simulink model "turbine_Drivetrain_modelling"  (R2024a)
settings: Solver=VariableStepAuto  StartTime=0.0  StopTime=200  MaxStep=0.4  RelTol=1e-3
model workspace (MAT data in the model file):
  para_mdl = Simulink.Parameter
  para_mdl.Value.N = 3
  para_mdl.Value.R = 63
  para_mdl.Value.rho = 1.225
  para_mdl.Value.mT = 436865
  para_mdl.Value.kT = 1981900
  para_mdl.Value.dT = 70000
  para_mdl.Value.rB = 21.975
  para_mdl.Value.mB = 4435
  para_mdl.Value.kB = 40000
  para_mdl.Value.kB_zentr = 0.02
  para_mdl.Value.dB = 20000
  para_mdl.Value.ngear = 97
  para_mdl.Value.Jr = 38759227
  para_mdl.Value.Jg = 534.1
  para_mdl.Value.kS = 92213.5189712
  para_mdl.Value.dS = 660.537782974
  para_mdl.Value.tau_beta = 0.1
  para_mdl.Value.betaP_max = 0.174532925199
  para_mdl.Value.tau_PT2 = 0.09
  para_mdl.Value.zeta_PT2 = 0.6
  para_mdl.Value.tau_g = 0.02
  para_mdl.Value.Tv = 4
  para_mdl.Value.Notch.om1 = 10.364
  para_mdl.Value.Notch.om2 = 8
  para_mdl.Value.Notch.zeta1 = 0.6
  para_mdl.Value.Notch.zeta2 = 1.2
  para_mdl.Value.Pr_R = 5296610
  para_mdl.Value.omega_r_R = 1.2671
  para_mdl.Value.omega_g_R = 122.9087
  para_mdl.Value.Tr_R = 4180104.17489
  para_mdl.Value.Tg_R = 43093.8574731
  para_mdl.Value.v_R = 11.26
  para_mdl.Value.J_1DOF = 43784573.9
  para_mdl.Value.CT_betas = [0 0.0872664625997 0.174532925199 0.261799387799 0.349065850399 0.436332312999 0.523598775598 0.698131700798 0.872664625997 1.0471975512 1.2217304764 1.3962634016 1.57079632679]
  para_mdl.Value.CT_lambdas = [0; 0.25; 0.5; 0.75; 1; 1.25; 1.5; 2; 2.5; 3; 3.5; 4; 4.5; 5; 5.5; 6; 6.5; 7; 7.5; 8; 8.5; 9; 9.5; 10; 10.5; 11; 11.5; 12; 12.5; 13; 13.5; 14; 14.5; 15; 15.5; 16; 16.5; 17; 17.5]
  para_mdl.Value.CQ_betas = [0 0.0872664625997 0.174532925199 0.261799387799 0.349065850399 0.436332312999 0.523598775598 0.698131700798 0.872664625997 1.0471975512 1.2217304764 1.3962634016 1.57079632679]
  para_mdl.Value.CQ_lambdas = [0; 0.25; 0.5; 0.75; 1; 1.25; 1.5; 2; 2.5; 3; 3.5; 4; 4.5; 5; 5.5; 6; 6.5; 7; 7.5; 8; 8.5; 9; 9.5; 10; 10.5; 11; 11.5; 12; 12.5; 13; 13.5; 14; 14.5; 15; 15.5; 16; 16.5; 17; 17.5]
  para_mdl.Value.CQ_entries = [0.00463492513935 0.0049015417371 0.00516815833485 0.00555696036228 0.0059457623897 0.00611397686765 0.00628219134561 0.012914252991 0.0255245334589 0.0349006692545 0.0430149587943 0.0524658396931 ... (507 elements, 39x13)]
  para_mdl.Value.CT_entries = [0.0686211548678 0.0728422059393 0.0770632570108 0.0836290674204 0.09019487783 0.0932108047116 0.0962267315932 0.135717354129 0.192838891055 0.239446349533 0.288110808378 0.351656989082 ... (507 elements, 39x13)]
  para_mdl.Value.Cp_max = 0.487647762952
  para_mdl.Value.lambda_opt = 7.5
  para_mdl.Complexity = 'real'
  para_mdl.Dimensions = [1 1]
  para_mdl.DataType = 'struct'
values from neighbouring files (symbols this model uses):
  beta = [0.0000, 0.0306, 0.0560, 0.0772, 0.0953, 0.1113, 0.1254, 0.1382,          0.1499, 0.1607, 0.1783, 0.2134, 0.2421, 0.2669, 0.2890, 0.3091,          0.3279, 0.3456, 0.3625, 0.3789]'    [Sensitivities.m]
  k_I = a./(b.*tau_ref)    [Sensitivities.m]
  k_P = 5./(b.*tau_ref)    [Sensitivities.m]
  para_mdl =     [para_mdl_WT_with_aero.mat]
  v = [11.2600, 11.5378, 11.8156, 12.0933, 12.3711, 12.6489, 12.9267,       13.2044, 13.4822, 13.7600, 14.2600, 15.4533, 16.6467, 17.8400,       19.0333, 20.2267, 21.4200, 22.6133, 23.8067, 25.0000]'    [Sensitivities.m]
settings Model: Creator=hasansinat  LastModifiedBy=Dell
settings SolverCC: AlgebraicLoopSolver=TrustRegion
settings RTWCC: GPUComputeCapability=3.5

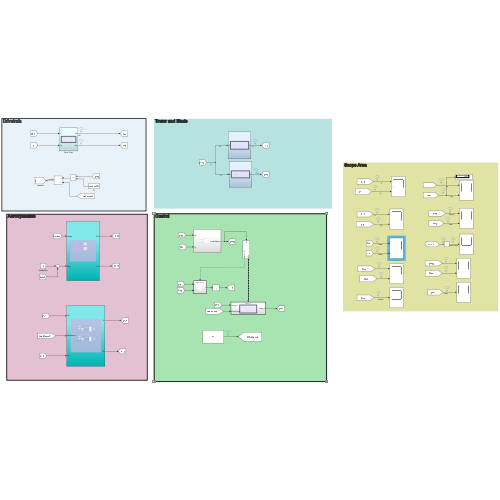
[thumbnail: Simulink's stored preview of the top-level diagram]
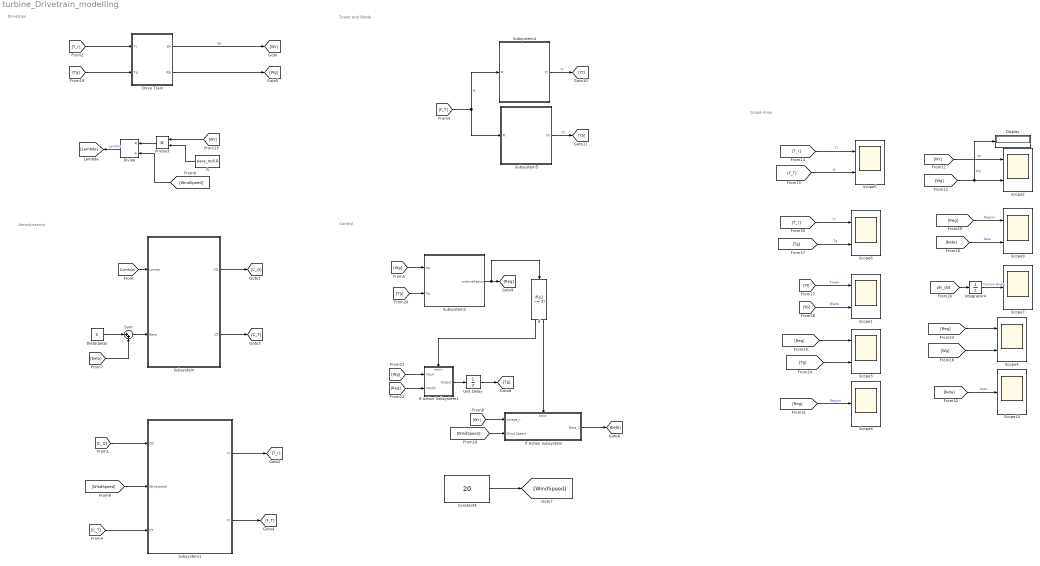
== system turbine_Drivetrain_modelling ==
  note: Aerodynamics
  note: Drivetrain
  note: Tower and Blade
  note: Control
  note: Scope Area
  Constant4 : Constant  Value=20
  Display : Display
  Divide : Product  Inputs=*/
  Drive Train : Subsystem
  If : If  IfExpression=u1 ~= 3
  If Action Subsystem : Subsystem  TreatAsAtomicUnit=on
  If Action Subsystem1 : Subsystem  TreatAsAtomicUnit=on
  Integrator4 : Integrator
  Product : Product
  R : Constant  Value=para_mdl.R
  Scope{1..6,9} (7 alike) : Scope  NumInputPorts=2
  Scope10 : Scope
  Scope7 : Scope
  Scope8 : Scope
  Subsystem : Subsystem
  Subsystem1 : Subsystem
  Subsystem2 : Subsystem
  Subsystem4 : Subsystem
  Subsystem5 : Subsystem
  Sum : Sum  Inputs=|++
  Unit Delay : UnitDelay  SampleTime=-1  HasFrameUpgradeWarning=on
  theta(beta) : Constant  Value=0
  wires:
  [T_r] -> Drive Train/1(Tr)
  Drive Train/1(Wr) -> [Wr]  "Wr"
  Product/1 -> Divide/1
  R/1 -> Product/2
  Divide/1 -> [Lambda]  "Lambda"
  Drive Train/2(Wg) -> [Wg]
  Unit Delay/1 -> [Tg]
  If/2 -> If Action Subsystem/Action
  If/1 -> If Action Subsystem1/Action
  If Action Subsystem/1(Beta_1) -> [beta]
  theta(beta)/1 -> Sum/1
  [Wr] -> If Action Subsystem/1(omega_r)
  [WindSpeed] -> If Action Subsystem/2(Wind Speed)
  [Wr] -> Scope2/1  "Wr"
  [Wg] -> Display/1, Scope2/2  "Wg"
  [Wr] -> Product/1
  [T_r] -> Scope5/1  "Tr"
  [F_T] -> Scope5/2  "Ft"
  [beta] -> Scope9/2  "beta"
  [Tg] -> Scope6/2  "Tg"
  [beta] -> Sum/2
  If Action Subsystem1/1(Output) -> Unit Delay/1
  [Wg] -> Scope4/2
  [Tg] -> Drive Train/2(Tg)
  [Wg] -> If Action Subsystem1/1(Input)
  [Reg] -> If Action Subsystem1/2(Input1)
  [Reg] -> Scope4/1
  [Tg] -> Scope3/2
  [Reg] -> Scope3/1
  [Lambda] -> Subsystem/1(Lamda)
  Sum/1 -> Subsystem/2(Beta)
  Subsystem/1(CQ) -> [C_Q]
  Subsystem/2(CT) -> [C_T]
  [C_Q] -> Subsystem1/1(CQ)
  [WindSpeed] -> Subsystem1/2(Windspeed)
  [C_T] -> Subsystem1/3(CT)
  Subsystem1/1(Tr) -> [T_r]
  Subsystem1/2(Ft) -> [F_T]
  Subsystem5/1(Yb) -> [Yb]  "Yb"
  [F_T] -> Subsystem5/1(Ft), Subsystem4/1(Ft)  "Ft"
  Subsystem4/1(Yt) -> [Yt]  "Yt"
  Subsystem2/1(turbineRegion) -> If/1, [Reg]
  [Wg] -> Subsystem2/1(wg)
  [Tg] -> Subsystem2/2(Tg)
  [phi_dot] -> Integrator4/1
  Integrator4/1 -> Scope7/1  "Torsion Angle"
  [Yb] -> Scope1/2  "Blade"
  [Yt] -> Scope1/1  "Tower"
  Constant4/1 -> [WindSpeed]
  [WindSpeed] -> Divide/2
  [Reg] -> Scope9/1  "Region"
  [T_r] -> Scope6/1  "Tr"
  [Reg] -> Scope8/1  "Region"
  [beta] -> Scope10/1  "beta"

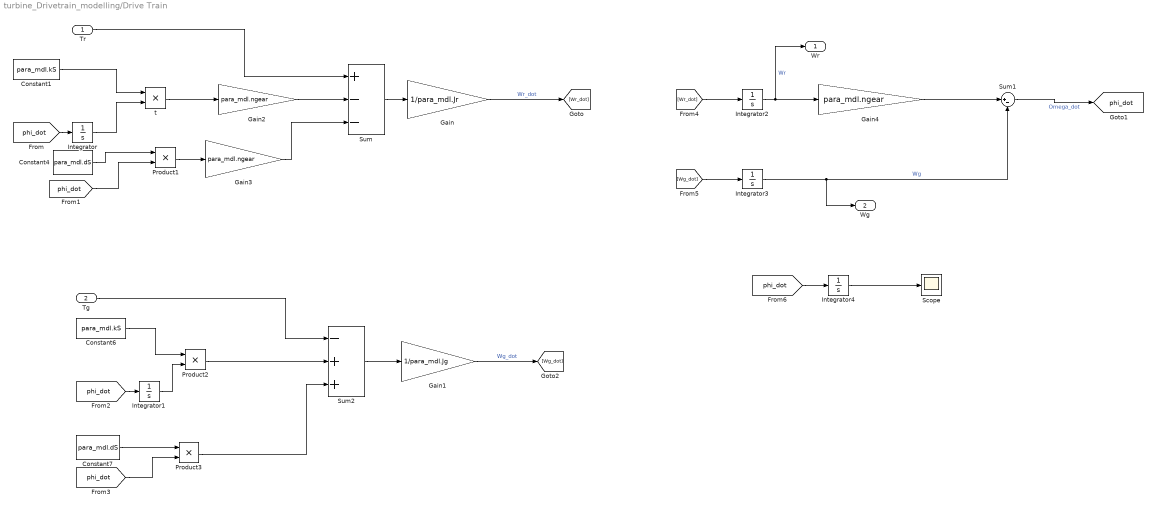
== system turbine_Drivetrain_modelling/Drive Train ==
  Tr : Inport
  Tg : Inport  Port=2
  Constant1 : Constant  Value=para_mdl.kS
  Constant4 : Constant  Value=para_mdl.dS
  Constant6 : Constant  Value=para_mdl.kS
  Constant7 : Constant  Value=para_mdl.dS
  Gain : Gain  Gain=1/para_mdl.Jr
  Gain1 : Gain  Gain=1/para_mdl.Jg
  Gain2 : Gain  Gain=para_mdl.ngear
  Gain3 : Gain  Gain=para_mdl.ngear
  Gain4 : Gain  Gain=para_mdl.ngear
  Integrator{,1..4} (5 alike) : Integrator
  Product1 : Product
  Product2 : Product
  Product3 : Product
  Scope : Scope
  Sum : Sum  Inputs=+--
  Sum1 : Sum  Inputs=|+-
  Sum2 : Sum  Inputs=-++
  t : Product
  Wr : Outport
  Wg : Outport  Port=2
  tag scope: phi_dot=global
  wires:
  [Wr_dot] -> Integrator2/1
  Gain4/1 -> Sum1/1
  [phi_dot] -> Integrator1/1
  Constant4/1 -> Product1/1
  Integrator2/1 -> Wr/1, Gain4/1  "Wr"
  Constant6/1 -> Product2/1
  Tg/1 -> Sum2/1
  Sum1/1 -> [phi_dot]  "Omega_dot"
  Constant7/1 -> Product3/1
  Integrator3/1 -> Wg/1, Sum1/2  "Wg"
  Sum/1 -> Gain/1
  Sum2/1 -> Gain1/1
  [phi_dot] -> Product3/2
  Gain1/1 -> [Wg_dot]  "Wg_dot"
  Constant1/1 -> t/1
  [phi_dot] -> Product1/2
  [phi_dot] -> Integrator/1
  Integrator1/1 -> Product2/2
  Integrator/1 -> t/2
  [Wg_dot] -> Integrator3/1
  Gain/1 -> [Wr_dot]  "Wr_dot"
  Tr/1 -> Sum/1
  t/1 -> Gain2/1
  Product2/1 -> Sum2/2
  Product3/1 -> Sum2/3
  Gain2/1 -> Sum/2
  Gain3/1 -> Sum/3
  [phi_dot] -> Integrator4/1
  Integrator4/1 -> Scope/1
  Product1/1 -> Gain3/1

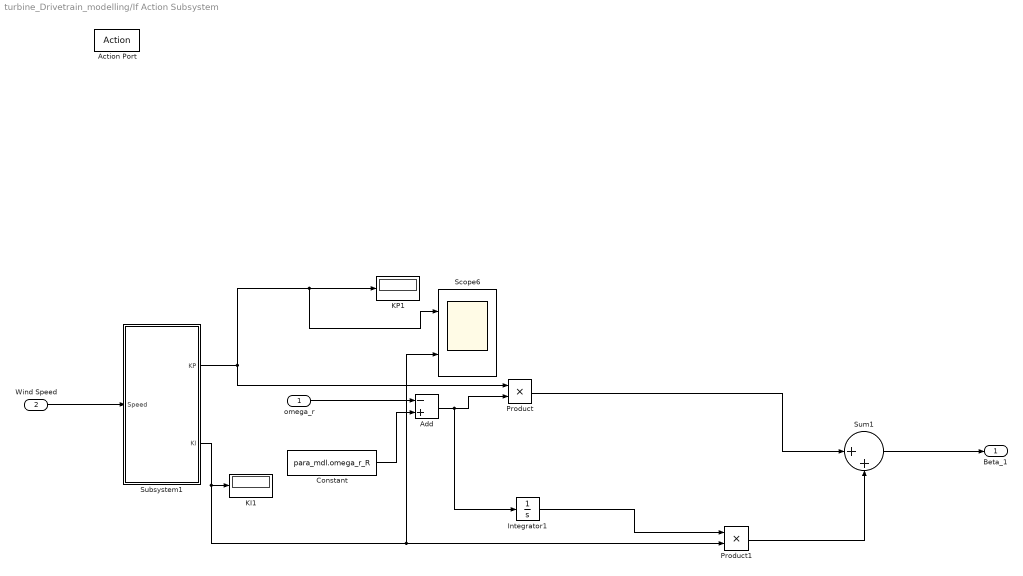
== system turbine_Drivetrain_modelling/If Action Subsystem ==
  omega_r : Inport
  Wind Speed : Inport  Port=2
  Action Port : ActionPort  ActionPortLabel=else
  Add : Sum  Inputs=-+
  Constant : Constant  Value=para_mdl.omega_r_R
  Integrator1 : Integrator
  KI1 : Display
  KP1 : Display
  Product : Product
  Product1 : Product
  Scope6 : Scope  NumInputPorts=2
  Subsystem1 : Subsystem  Priority=1
  Sum1 : Sum  Inputs=|++
  Beta_1 : Outport
  wires:
  Constant/1 -> Add/2
  Integrator1/1 -> Product1/1
  Add/1 -> Integrator1/1, Product/2
  Product/1 -> Sum1/1
  Wind Speed/1 -> Subsystem1/1(Speed)
  Sum1/1 -> Beta_1/1
  Subsystem1/2(" KI") -> Scope6/2, Product1/2, KI1/1
  Subsystem1/1(" KP") -> Scope6/1, KP1/1, Product/1
  omega_r/1 -> Add/1
  Product1/1 -> Sum1/2

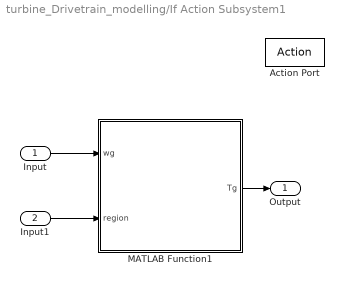
== system turbine_Drivetrain_modelling/If Action Subsystem1 ==
  Input : Inport
  Input1 : Inport  Port=2
  Action Port : ActionPort  ActionPortLabel=if(u1 ~= 3)
  MATLAB Function1 : MATLAB Function  TreatAsAtomicUnit=on
  Output : Outport
  wires:
  Input1/1 -> MATLAB Function1/2(region)
  Input/1 -> MATLAB Function1/1(wg)
  MATLAB Function1/1(Tg) -> Output/1

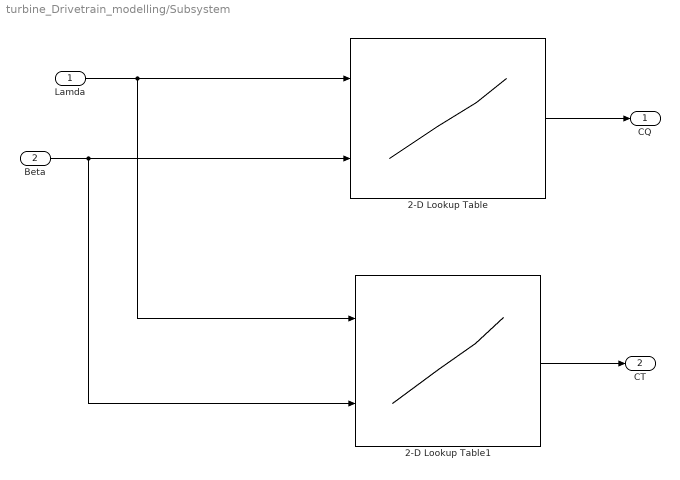
== system turbine_Drivetrain_modelling/Subsystem ==
  Lamda : Inport
  Beta : Inport  Port=2
  2-D Lookup Table : Lookup_n-D  BreakpointsForDimension1=para_mdl.CQ_lambdas  BreakpointsForDimension2=para_mdl.CQ_betas  Table=para_mdl.CQ_entries  InternalRulePriority=Speed  RndMeth=Simplest
      settings: InputPortMap=u0,u1
  2-D Lookup Table1 : Lookup_n-D  BreakpointsForDimension1=para_mdl.CT_lambdas  BreakpointsForDimension2=para_mdl.CT_betas  Table=para_mdl.CT_entries  InternalRulePriority=Speed  RndMeth=Simplest
      settings: InputPortMap=u0,u1
  CQ : Outport
  CT : Outport  Port=2
  wires:
  Beta/1 -> 2-D Lookup Table/2, 2-D Lookup Table1/2
  2-D Lookup Table1/1 -> CT/1
  Lamda/1 -> 2-D Lookup Table1/1, 2-D Lookup Table/1
  2-D Lookup Table/1 -> CQ/1

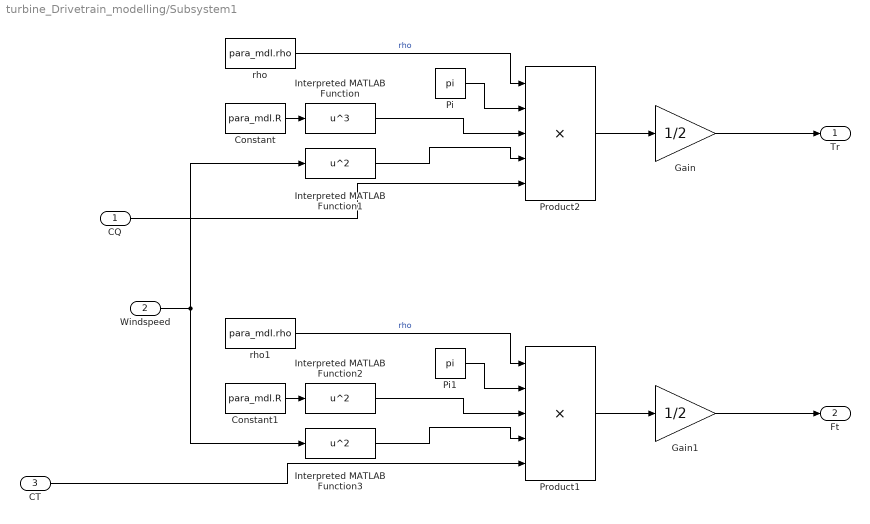
== system turbine_Drivetrain_modelling/Subsystem1 ==
  CQ : Inport
  Windspeed : Inport  Port=2
  CT : Inport  Port=3
  Constant : Constant  Value=para_mdl.R
  Constant1 : Constant  Value=para_mdl.R
  Gain : Gain  Gain=1/2
  Gain1 : Gain  Gain=1/2
  Interpreted MATLAB Function : MATLABFcn  MATLABFcn=u^3
  Interpreted MATLAB Function1 : MATLABFcn  MATLABFcn=u^2
  Interpreted MATLAB Function2 : MATLABFcn  MATLABFcn=u^2
  Interpreted MATLAB Function3 : MATLABFcn  MATLABFcn=u^2
  Pi : Constant  Value=pi  OutDataTypeStr=Inherit: Inherit via back propagation
  Pi1 : Constant  Value=pi  OutDataTypeStr=Inherit: Inherit via back propagation
  Product1 : Product  Inputs=5
  Product2 : Product  Inputs=5
  rho : Constant  Value=para_mdl.rho
  rho1 : Constant  Value=para_mdl.rho
  Tr : Outport
  Ft : Outport  Port=2
  wires:
  Product2/1 -> Gain/1
  Windspeed/1 -> Interpreted MATLAB Function1/1, Interpreted MATLAB Function3/1
  Product1/1 -> Gain1/1
  Pi/1 -> Product2/2
  Interpreted MATLAB Function1/1 -> Product2/4
  Pi1/1 -> Product1/2
  Interpreted MATLAB Function3/1 -> Product1/4
  Gain/1 -> Tr/1
  Constant/1 -> Interpreted MATLAB Function/1
  Gain1/1 -> Ft/1
  Constant1/1 -> Interpreted MATLAB Function2/1
  Interpreted MATLAB Function2/1 -> Product1/3
  rho/1 -> Product2/1  "rho"
  Interpreted MATLAB Function/1 -> Product2/3
  rho1/1 -> Product1/1  "rho"
  CQ/1 -> Product2/5
  CT/1 -> Product1/5

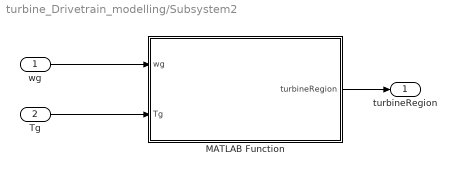
== system turbine_Drivetrain_modelling/Subsystem2 ==
  wg : Inport
  Tg : Inport  Port=2
  MATLAB Function : MATLAB Function  TreatAsAtomicUnit=on
  turbineRegion : Outport
  wires:
  wg/1 -> MATLAB Function/1(wg)
  Tg/1 -> MATLAB Function/2(Tg)
  MATLAB Function/1(turbineRegion) -> turbineRegion/1

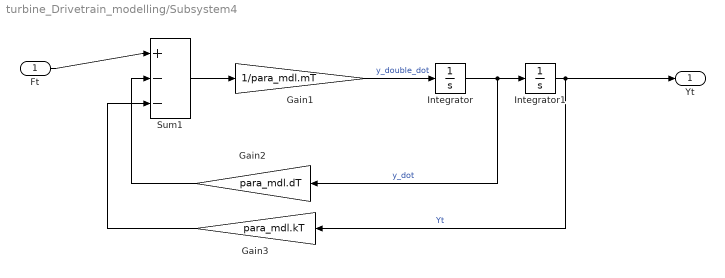
== system turbine_Drivetrain_modelling/Subsystem4 ==
  Ft : Inport
  Gain1 : Gain  Gain=1/para_mdl.mT
  Gain2 : Gain  Gain=para_mdl.dT
  Gain3 : Gain  Gain=para_mdl.kT
  Integrator : Integrator
  Integrator1 : Integrator
  Sum1 : Sum  Inputs=|+--
  Yt : Outport
  wires:
  Sum1/1 -> Gain1/1
  Ft/1 -> Sum1/1
  Integrator1/1 -> Yt/1, Gain3/1  "Yt"
  Gain2/1 -> Sum1/2
  Gain1/1 -> Integrator/1  "y_double_dot"
  Gain3/1 -> Sum1/3
  Integrator/1 -> Integrator1/1, Gain2/1  "y_dot"

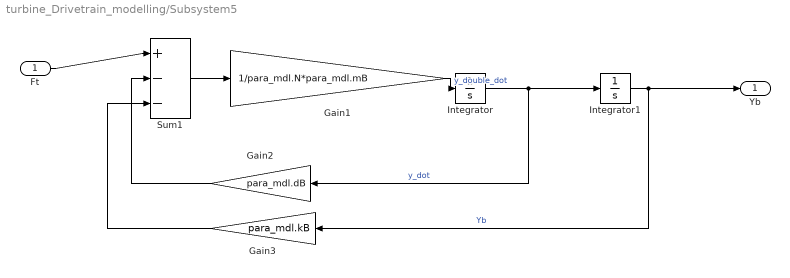
== system turbine_Drivetrain_modelling/Subsystem5 ==
  Ft : Inport
  Gain1 : Gain  Gain=1/para_mdl.N*para_mdl.mB
  Gain2 : Gain  Gain=para_mdl.dB
  Gain3 : Gain  Gain=para_mdl.kB
  Integrator : Integrator
  Integrator1 : Integrator
  Sum1 : Sum  Inputs=|+--
  Yb : Outport
  wires:
  Integrator/1 -> Integrator1/1, Gain2/1  "y_dot"
  Gain3/1 -> Sum1/3
  Gain1/1 -> Integrator/1  "y_double_dot"
  Gain2/1 -> Sum1/2
  Integrator1/1 -> Yb/1, Gain3/1  "Yb"
  Ft/1 -> Sum1/1
  Sum1/1 -> Gain1/1

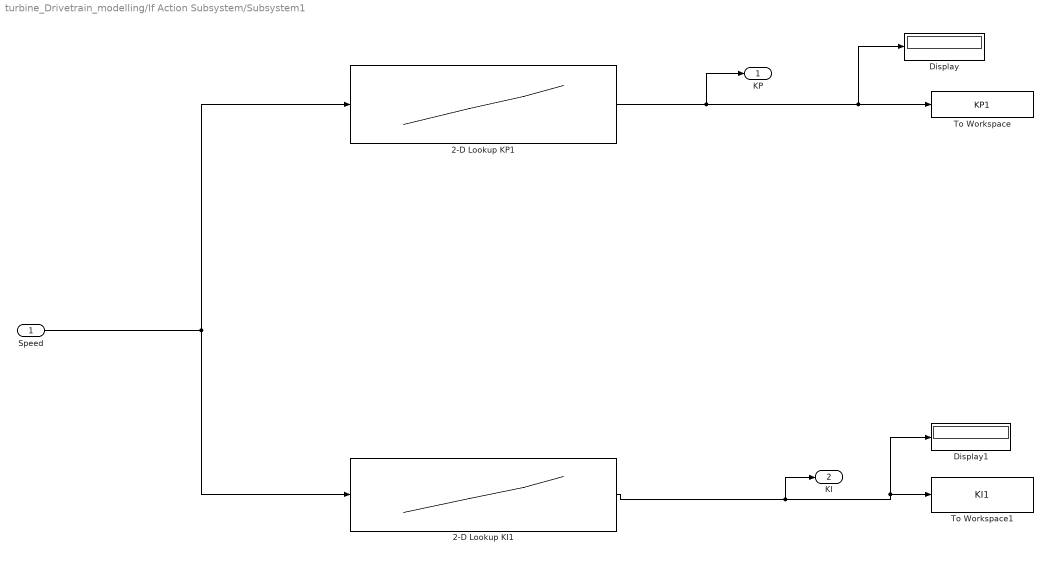
== system turbine_Drivetrain_modelling/If Action Subsystem/Subsystem1 ==
  Speed : Inport
  2-D Lookup KI1 : Lookup_n-D  NumberOfTableDimensions=1  BreakpointsForDimension1=v  BreakpointsForDimension2=beta  Table=k_I  InternalRulePriority=Speed  RndMeth=Simplest
  2-D Lookup KP1 : Lookup_n-D  NumberOfTableDimensions=1  BreakpointsForDimension1=v  BreakpointsForDimension2=[1:3]  Table=k_P  InternalRulePriority=Speed  RndMeth=Simplest
  Display : Display
  Display1 : Display
  To Workspace : ToWorkspace  VariableName=KP1  SaveFormat=Timeseries  SampleTime=-1
  To Workspace1 : ToWorkspace  VariableName=KI1  SaveFormat=Timeseries  SampleTime=-1
  " KP" : Outport
  " KI" : Outport  Port=2
  wires:
  2-D Lookup KI1/1 -> " KI"/1, Display1/1, To Workspace1/1
  Speed/1 -> 2-D Lookup KP1/1, 2-D Lookup KI1/1
  2-D Lookup KP1/1 -> " KP"/1, Display/1, To Workspace/1

== matlab function turbine_Drivetrain_modelling/Subsystem2/MATLAB Function ==
  settings: updateMethod=DISCRETE
  data: wg input; turbineRegion output; Tg input
function turbineRegion = fcn(wg, Tg)
    %#codegen

    % Define the thresholds for the conditions
    wg_rated = 1.229087000000000e+02;
    wg_R1_max = wg_rated * 0.5708; 
    wg_R1_5_max = wg_rated * 0.7421;
    wg_R2_max = wg_rated * 0.9782;
    wg_R2_5_max = wg_rated * 0.99;
     
    dwg = 2;
    Tg_max = 4.309385747306741e+04;

    % Define a persistent variable to store the previous region
    persistent prev_region
    if isempty(prev_region)
        prev_region = 1; % initialize with the starting region
    end
    % Declare that prev_region can have a variable size
    coder.varsize('prev_region', [1, 5], [0, 1]); % [1, 5] is the maximum size, [0, 1] indicates that the second dimension can vary

    % Initialize the region output
    turbineRegion = 0;
    % Check the conditions for each region
    switch prev_region
        case 1 % Region_1
            if wg > wg_R1_max
                turbineRegion = 1.5; % Region_1.5
            else
                turbineRegion = 1; % Region_1
            end
        case 2 % Region_1.5
            if wg > wg_R1_5_max
                turbineRegion = 2; % Region_2
            elseif wg <= wg_R1_max
                turbineRegion = 1; % Region_1
            else
                turbineRegion = 1.5; % Region_1.5
            end
        case 3 % Region_2
            if wg > wg_R2_max && Tg > Tg_max
                turbineRegion = 2.5; % Region_2.5
            elseif wg <= wg_R1_5_max
                turbineRegion = 1.5; % Region_1.5
            else
                turbineRegion = 2; % Region_2
            end
        case 4 % Region_2.5
            if wg > wg_R2_5_max && Tg > Tg_max
                turbineRegion = 3; % Region_3
            elseif wg <= (wg_R2_max - dwg)
                turbineRegion = 2; % Region_2
            else
                turbineRegion = 2.5; % Region_2.5
            end
        case 5 % Region_3
            if wg <= wg_R2_5_max || Tg <= Tg_max
                turbineRegion = 2.5; % Region_2.5
            else
                turbineRegion = 3; % Region_3
            end
    end

    % Update the previous region
    prev_region = find([1, 1.5, 2, 2.5, 3] == turbineRegion);
end

== matlab function turbine_Drivetrain_modelling/If Action Subsystem1/MATLAB Function1 ==
  data: wg input; Tg output; region input
function Tg = calculateTg(wg, region)
    % Calculation for Tg based on operating region

    wg_rated = 1.229087000000000e+02;
    Tg_max = 4.309385747306741e+04;
    k_Opt = 2.418610624349642;
    %k_Opt = 0.5 * 1.2250 * pi * 63^5 * (0.4876/(97^3*7.5^3)) * wg^2;
    
    switch region
        case 1
            Tg = 0; % Region 1
        case 1.5
            Tg = (3*(wg/wg_rated) - 1.8)*Tg_max; % Region 1.5
        case 2
            Tg = k_Opt * wg^2; % Region 2
        case 2.5
            Tg = (5.5*(wg/wg_rated) - 4.61)*Tg_max; % Region 2.5
        otherwise
            Tg = 0; % Default value for other regions
    end
end
